simulink model "Weir_aerator"  (Simulink 7.9)
settings: Solver=ode15s  StartTime=0.0  StopTime=24*3600  MaxStep=1000  RelTol=1e-5  AbsTol=1e-5
undefined symbols (not defined in the file or in its folder): B, U, x0
settings Model: Creator=psross  LastModifiedBy=M.Sparnaaij  ExtModeTrigMode=oneshot  ExtModeArmWhenConnect=off
settings DataIOCC: LimitDataPoints=off  SaveOutput=off  SaveTime=off  SignalLoggingName=sigsOut
settings OptimizationCC: BooleanDataType=off
settings DebuggingCC: SaveWithParameterizedLinksMsg=none  SignalResolutionControl=TryResolveAllWithWarning  SolverPrmCheckMsg=none  MultiTaskDSMMsg=warning  MultiTaskCondExecSysMsg=none  FcnCallInpInsideContextMsg=Use local settings  StrictBusMsg=None
settings HardwareCC: TargetUnknown=on
settings RTWCC: IncludeERTFirstTime=on
settings GRTTargetCC: CombineOutputUpdateFcns=off  GRTInterface=on

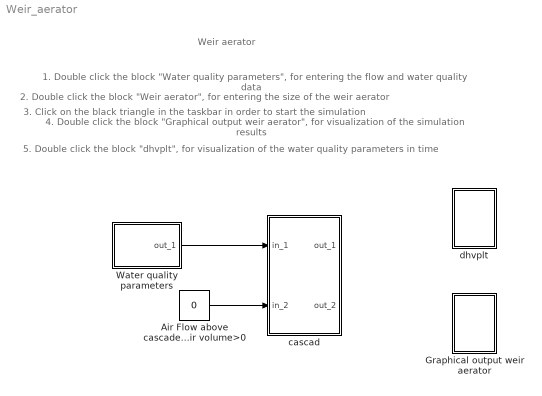
== system Weir_aerator ==
  note: 1. Double click the block "Water quality parameters", for entering the flow and water quality data
  note: 2. Double click the block "Weir aerator", for entering the size of the weir aerator
  note: 3. Click on the black triangle in the taskbar in order to start the simulation
  note: 4. Double click the block "Graphical output weir aerator", for visualization of the simulation results
  note: Weir aerator
  note: 5. Double click the block "dhvplt", for visualization of the water quality parameters in time
  Air Flow above cascade if air volume>0 : Constant  Value=0
  Graphical output weir aerator : Subsystem
      settings: OpenFcn=cascad_g
      mask Display:
      | plot(0,0,100,100,[80,20,20],[20,20,80],[80,69,60,52,45,39,33,28,24,20],[65,65,64,61,57,52,45,37,30,20])
      | disp('');
      | text(100,100,'cascad', 'horizontalAlignment', 'right', 'verticalAlignment', 'top');
  Water quality parameters : Subsystem  Description=The water flow and the water quality data must be filled out in the 'Water quality parameters' block. Each project must start with a 'Water quality parameters' block.
      mask init:
      | filenaam='./StimelaData/Water_qual_param.mat';
      | 
      | [Pn,Fn,Fext]=Fileprop(filenaam);
      | 
      | errstr = st_UniqName(filenaam,'filenaam=''','SubSystem','OpenFcn');
      | if errstr, error([errstr 'The filename "' filenaam '" is already in use. Choose a different filename.']), end
      | 
      | P = invruw_p(filenaam);
      | [B,x0,U]=invruw_i(filenaam);
      settings: OpenFcn=|
      | filenaam='./StimelaData/Water_qual_param.mat';
      | st_ParameterInput('init',gcb,filenaam,'invruw');
      mask Display:
      | plot(0,0,100,100,[80 100],[ 50 50],[80 100],[ 55 55],[20 80 80 20 20],[10 10 90  90 10]);
      | disp('')
      | text(50,50,'invruw', 'horizontalAlignment', 'center', 'verticalAlignment', 'middle');
      | text(50,0,Fn, 'horizontalAlignment', 'center', 'verticalAlignment', 'base');
  cascad : Subsystem  Description=This model calculates the aeration and degassifying with a weir aerator. The influent carbon dioxide concentration is calculated on the basis of the bicarbonate concentration, the pH, the EGV and the water temperature, so these parameters must always be filled out in the 'Water quality parameters' block.
      mask init:
      | filenaam='./StimelaData/Weir_aerator.mat';
      | 
      | [Pn,Fn,Fext]=Fileprop(filenaam);
      | 
      | errstr = st_UniqName(filenaam,'filenaam=''','SubSystem','OpenFcn');
      | if errstr, error([errstr 'The filename "' filenaam '" is already in use. Choose a different filename.']), end
      | 
      | P = cascad_p(filenaam);
      | [B,x0,U]=cascad_i(filenaam);
      settings: OpenFcn=|
      | filenaam='./StimelaData/Weir_aerator.mat';
      | st_ParameterInput('init',gcb,filenaam,'cascad');
      mask Display:
      | plot(0,0,100,100,[40,40,20,20],[80,60,60,80],[60,60,40,40],[60,40,40,60],[80,80,60,60],[40,20,20,40],[50,49,48,46,44,40],[60,66,71,76,79,80],[45,45,44,43,41,40],[60,66,71,75,78,80],[70,69,68,66,64,60],[40,48,53,57,59,61],[65,65,64,63,62,60],[40,45,51,55,58,60],[40,20],[80,80],[60,40],[60,60],[80,60],[40,40])
      | disp('')
      | text(50,50,'cascad', 'horizontalAlignment', 'center', 'verticalAlignment', 'middle');
      | text(50,0,Fn, 'horizontalAlignment', 'center', 'verticalAlignment', 'base');
  dhvplt : Subsystem
      settings: OpenFcn=plotStimela2
      mask Display:
      | plot(0,0,100,100,[80,20,20],[20,20,80],[80,69,60,52,45,39,33,28,24,20],[65,65,64,61,57,52,45,37,30,20])
      | disp('');
      | text(100,100,'Stimela', 'horizontalAlignment', 'right', 'verticalAlignment', 'top');
  wires:
  Water quality parameters/1(out_1) -> cascad/1(in_1)
  Air Flow above cascade if air volume>0/1 -> cascad/2(in_2)

== system Weir_aerator/Graphical output weir aerator ==
  note: plotten

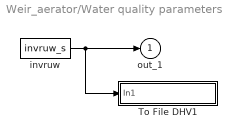
== system Weir_aerator/Water quality parameters ==
  To File DHV1 : Subsystem  mask(To File DHV){naam=[filenaam(1:length(filenaam)-4) '_out.sti']}
      mask prompts: naam "Naam van bestand"
      mask init:
      | set_param([gcb '/To File'],'Filename',naam);
      mask Display: disp(naam)
  invruw : S-Function  FunctionName=invruw_s  Parameters=B,x0,U,P  EnableBusSupport=off
  out_1 : Outport  InitialOutput=0
  wires:
  invruw/1 -> out_1/1, To File DHV1/1(In1)

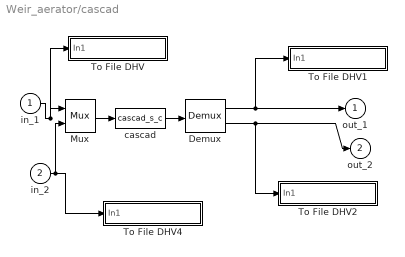
== system Weir_aerator/cascad ==
  in_1 : Inport
  in_2 : Inport  Port=2
  Demux : Demux  Outputs=[U.Number B.Measurements]
  Mux : Mux  Inputs=[U.Number B.Setpoints]
  To File DHV : Subsystem  mask(To File DHV){naam=[filenaam(1:length(filenaam)-4) '_in.sti']}
      mask prompts: naam "Naam van bestand"
      mask init:
      | set_param([gcb '/To File'],'Filename',naam);
      mask Display: disp(naam)
  To File DHV1 : Subsystem  mask(To File DHV){naam=[filenaam(1:length(filenaam)-4) '_out.sti']}
      mask prompts: naam "Naam van bestand"
      mask init:
      | set_param([gcb '/To File'],'Filename',naam);
      mask Display: disp(naam)
  To File DHV2 : Subsystem  mask(To File DHV){naam=[filenaam(1:length(filenaam)-4) '_EM.sti']}
      mask prompts: naam "Naam van bestand"
      mask init:
      | set_param([gcb '/To File'],'Filename',naam);
      mask Display: disp(naam)
  To File DHV4 : Subsystem  mask(To File DHV){naam=[filenaam(1:length(filenaam)-4) '_ES.sti']}
      mask prompts: naam "Naam van bestand"
      mask init:
      | set_param([gcb '/To File'],'Filename',naam);
      mask Display: disp(naam)
  cascad : S-Function  FunctionName=cascad_s_c  Parameters=B,x0,U,P  EnableBusSupport=off
  out_1 : Outport  InitialOutput=0
  out_2 : Outport  Port=2  InitialOutput=0
  wires:
  Mux/1 -> cascad/1
  in_2/1 -> Mux/2, To File DHV4/1(In1)
  cascad/1 -> Demux/1
  Demux/1 -> out_1/1, To File DHV1/1(In1)
  Demux/2 -> out_2/1, To File DHV2/1(In1)
  in_1/1 -> Mux/1, To File DHV/1(In1)

== system Weir_aerator/dhvplt ==
  note: plotten

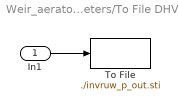
== system Weir_aerator/Water quality parameters/To File DHV1 ==
  In1 : Inport
  To File : ToFile  Filename=./invruw_p_out.sti  MatrixName=invruwout
  wires:
  In1/1 -> To File/1

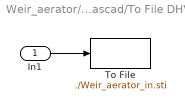
== system Weir_aerator/cascad/To File DHV ==
  In1 : Inport
  To File : ToFile  Filename=./Weir_aerator_in.sti  MatrixName=cascadin
  wires:
  In1/1 -> To File/1

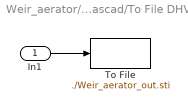
== system Weir_aerator/cascad/To File DHV1 ==
  In1 : Inport
  To File : ToFile  Filename=./Weir_aerator_out.sti  MatrixName=cascadout
  wires:
  In1/1 -> To File/1

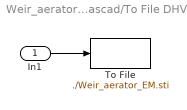
== system Weir_aerator/cascad/To File DHV2 ==
  In1 : Inport
  To File : ToFile  Filename=./Weir_aerator_EM.sti  MatrixName=cascadEM
  wires:
  In1/1 -> To File/1

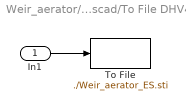
== system Weir_aerator/cascad/To File DHV4 ==
  In1 : Inport
  To File : ToFile  Filename=./Weir_aerator_ES.sti  MatrixName=cascadES
  wires:
  In1/1 -> To File/1
